simulink model "abe_x_theta_simple_R2021a"  (R2021a)
settings: Solver=VariableStepAuto  StartTime=0.0  StopTime=50  RelTol=1e-3
libraries: simulink x1
settings Model: Creator=Abraham  LastModifiedBy=Abraham
settings DebuggingCC: UnconnectedInputMsg=none  UnconnectedOutputMsg=none  UnconnectedLineMsg=none
settings RTWCC: DLArmComputeVersion=20.02.1

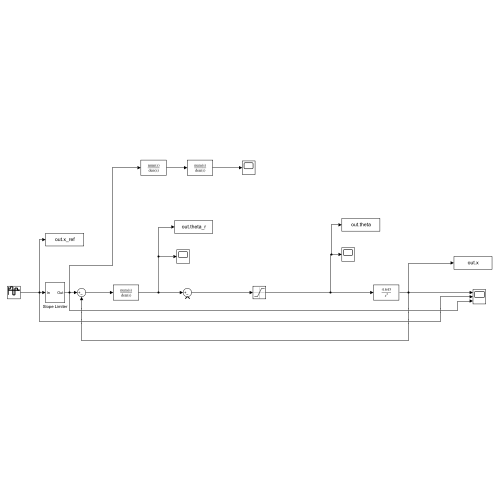
[thumbnail: Simulink's stored preview of the top-level diagram]
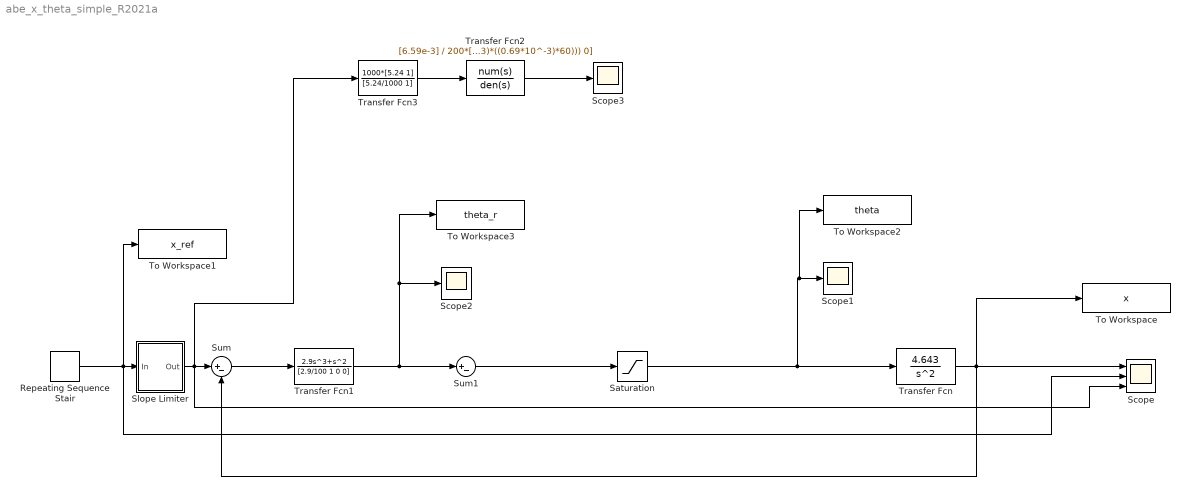
== system abe_x_theta_simple_R2021a ==
  Repeating Sequence Stair : simulink/Sources/Repeating Sequence Stair  OutValues=[5 15 -20 10 0]  tsamp=10  OutMin=[]  OutMax=[]  OutDataTypeStr=double  OutputDataTypeScalingMode=double  OutDataType=fixdt(0,8)  ConRadixGroup=Best Precision: Vector-wise  OutScaling=2^-12
  Saturation : Saturate  UpperLimit=6  LowerLimit=-6
  Scope : Scope  NumInputPorts=3
  Scope1 : Scope
  Scope2 : Scope
  Scope3 : Scope
  Slope Limiter : Subsystem
  Sum : Sum  Inputs=|+-
  Sum1 : Sum  Inputs=|+-
  To Workspace : ToWorkspace  VariableName=x  SaveFormat=Timeseries  SampleTime=-1
  To Workspace1 : ToWorkspace  VariableName=x_ref  SaveFormat=Timeseries  SampleTime=-1
  To Workspace2 : ToWorkspace  VariableName=theta  SaveFormat=Timeseries  SampleTime=-1
  To Workspace3 : ToWorkspace  VariableName=theta_r  SaveFormat=Timeseries  SampleTime=-1
  Transfer Fcn : TransferFcn  Numerator=[4.643]  Denominator=[1 0 0]
  Transfer Fcn1 : TransferFcn  Numerator=[2.9 1 0 0]  Denominator=[2.9/100 1 0 0]
  Transfer Fcn2 : TransferFcn  Numerator=[6.59e-3]  Denominator=200*[((75e-6)*(1e-7)) ((75e-6)*(1.67e-5)+(3.41*1e-7)) ((3.41*1.67e-5)+((6.59e-3)*((0.69*10^-3)*60))) 0]
  Transfer Fcn3 : TransferFcn  Numerator=1000*[5.24 1]  Denominator=[5.24/1000 1]
  wires:
  Transfer Fcn/1 -> To Workspace/1, Scope/1, Sum/2
  Slope Limiter/1(Out) -> Scope/3, Transfer Fcn3/1, Sum/1
  Repeating Sequence Stair/1 -> To Workspace1/1, Scope/2, Slope Limiter/1(In)
  Sum/1 -> Transfer Fcn1/1
  Transfer Fcn1/1 -> To Workspace3/1, Scope2/1, Sum1/1
  Saturation/1 -> To Workspace2/1, Scope1/1, Transfer Fcn/1
  Sum1/1 -> Saturation/1
  Transfer Fcn3/1 -> Transfer Fcn2/1
  Transfer Fcn2/1 -> Scope3/1

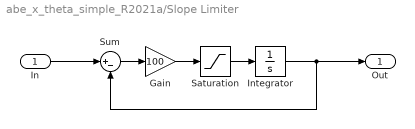
== system abe_x_theta_simple_R2021a/Slope Limiter ==
  In : Inport
  Gain : Gain  Gain=100
  Integrator : Integrator
  Saturation : Saturate  UpperLimit=10  LowerLimit=-10
  Sum : Sum  Inputs=|+-
  Out : Outport
  wires:
  Integrator/1 -> Out/1, Sum/2
  Gain/1 -> Saturation/1
  Saturation/1 -> Integrator/1
  Sum/1 -> Gain/1
  In/1 -> Sum/1
